simulink model "roughslx"  (R2015a)
settings: Solver=ode45  StartTime=0.0  StopTime=10.0  RelTol=1e-3
libraries: simulink x2
settings Model: Creator=admin  LastModifiedBy=admin

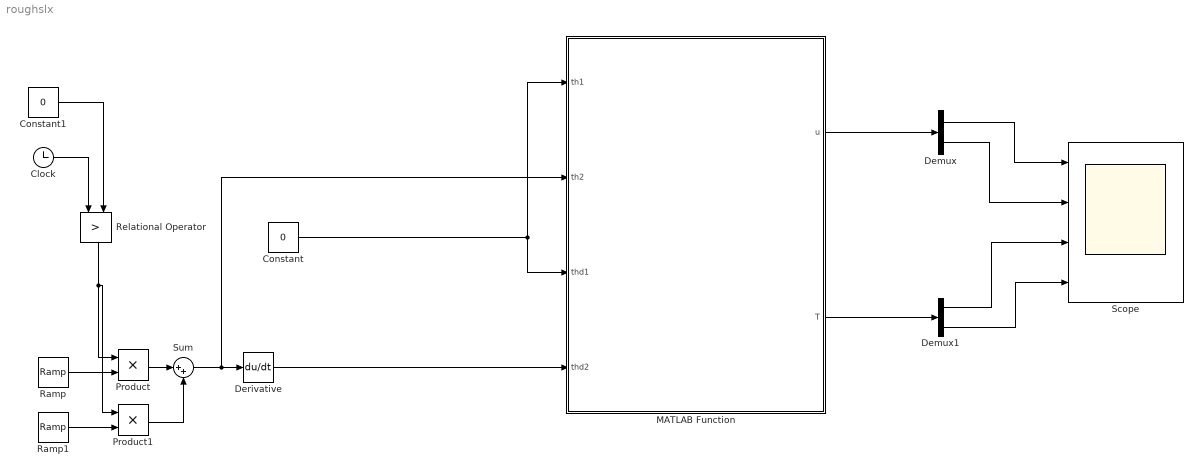
== system roughslx ==
  Clock : Clock
  Constant : Constant  Value=0
  Constant1 : Constant  Value=0
  Demux : Demux  Outputs=2
  Demux1 : Demux  Outputs=2
  Derivative : Derivative
  MATLAB Function : MATLAB Function  TreatAsAtomicUnit=on
  Product : Product
  Product1 : Product
  Ramp : simulink/Sources/Ramp  slope=1  start=1  X0=0
  Ramp1 : simulink/Sources/Ramp  slope=-1  start=8  X0=0
  Relational Operator : RelationalOperator  Operator=>  OutDataTypeStr=boolean
  Scope : Scope  NumInputPorts=4
      settings: YMin=-500~-1~-50~-5  YMax=2~1~50~5
  Sum : Sum  Inputs=|++
  wires:
  MATLAB Function/1(u) -> Demux/1
  Demux/1 -> Scope/1
  Demux/2 -> Scope/2
  MATLAB Function/2(T) -> Demux1/1
  Demux1/1 -> Scope/3
  Demux1/2 -> Scope/4
  Derivative/1 -> MATLAB Function/4(thd2)
  Sum/1 -> MATLAB Function/2(th2), Derivative/1
  Constant/1 -> MATLAB Function/1(th1), MATLAB Function/3(thd1)
  Clock/1 -> Relational Operator/1
  Constant1/1 -> Relational Operator/2
  Ramp/1 -> Product/2
  Relational Operator/1 -> Product1/1, Product/1
  Product/1 -> Sum/1
  Ramp1/1 -> Product1/2
  Product1/1 -> Sum/2

== matlab function roughslx/MATLAB Function ==
  data: u output; T output; th1 input; th2 input; thd1 input; thd2 input
function [u,T] = fcn(th1,th2,thd1,thd2)
%% Script file to simulate with parameters
K = [    1.0000         0       1.7321         0;
         0          1.0000         0        1.7321];
a1 = 0.20;
a2 = 0.40;
m1 = 2;
m2 = 2;
g = 9.8;
%intial conditions
u = -K*[th1;th2;thd1;thd2];
u1 = u(1);
u2 = u(2);
T = [(g*(a1*m1*cos(th1) + 2*a1*m2*cos(th1) + a2*m2*cos(th1 + th2)))/2 + (thd1 - u1)*((a1^2*m1)/3 + a1^2*m2 + (a2^2*m2)/3 + a1*a2*m2*cos(th2)) + (a2*m2*(thd2 - u2)*(2*a2 + 3*a1*cos(th2)))/6 - (a1*a2*m2*thd2*sin(th2)*(2*thd1 + thd2))/2;
                                                                                                   (a2^2*m2*(thd2 - u2))/3 + (a2*g*m2*cos(th1 + th2))/2 + (a2*m2*(thd1 - u1)*(2*a2 + 3*a1*cos(th2)))/6 + (a1*a2*m2*thd1^2*sin(th2))/2];
end
